simulink model "one_bot_form1"  (R2016b)
settings: Solver=ode3  StartTime=0.0  StopTime=1000  FixedStep=0.2  RelTol=1e-3  EnableMultiTasking=on
undefined symbols (not defined in the file): Angular, Linear
libraries: robotlib x7, simulink x6, realtime_pacer_lib x2
settings Model: Creator=The MathWorks Inc.  LastModifiedBy=esther
settings DataIOCC: LimitDataPoints=on  SaveFormat=Array
settings OptimizationCC: LifeSpan=Inf  MaxStackSize=64
settings DebuggingCC: SolverPrmCheckMsg=warning  SFUnexpectedBacktrackingDiag=warning  SFNoUnconditionalDefaultTransitionDiag=warning  SFExecutionAtInitializationDiag=none
settings HardwareCC: ProdBitPerPointer=32  ProdBitPerSizeT=32  ProdBitPerPtrDiffT=32  ProdLargestAtomicFloat=None  ProdIntDivRoundTo=Undefined  ProdEndianess=Unspecified  ProdWordSize=32  ProdHWDeviceType=Generic->Unspecified (assume 32-bit Generic)  TargetHWDeviceType=Generic->Unspecified (assume 32-bit Generic)
settings ModelReferenceCC: PropagateSignalLabelsOutOfModel=off
settings RTWCC: SystemTargetFile=ert.tlc  HardwareBoard=Robot Operating System (ROS)  TLCOptions=-aInlineSetEventsForThisBaseRateFcn=TLC_FALSE -aSuppressMultiTaskScheduler=TLC_FALSE -aRateBasedStepFcn=0  TemplateMakefile=ert_default_tmf  Description=Embedded Coder  Toolchain=Catkin  TargetLang=C++
settings ERTTargetCC: MultiInstanceERTCode=on  CodeInterfacePackaging=C++ class  SupportContinuousTime=on  RootIOFormat=Structure reference  ConvertIfToSwitch=off  SuppressUnreachableDefaultCases=off
settings ConfigComp: CovMetricSettings=dw  CovHtmlReporting=on  CovSaveCumulativeToWorkspaceVar=on  CovSaveSingleToWorkspaceVar=on  CovExternalEMLEnable=off  CovSFcnEnable=off

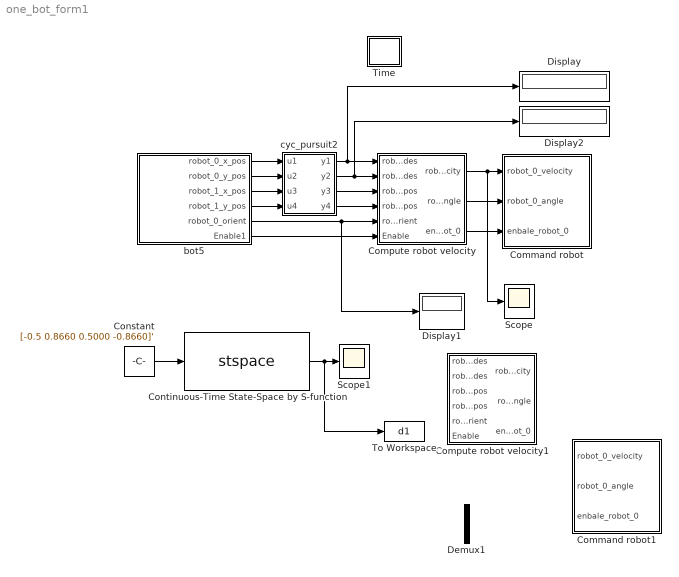
== system one_bot_form1 ==
  Command robot : Subsystem
  Command robot1 : Subsystem
  Compute robot velocity : Subsystem
  Compute robot velocity1 : Subsystem
  Constant : Constant  Value=[-0.5 0.8660 0.5000 -0.8660]'  SampleTime=-1
  Continuous-Time State-Space by S-function : S-Function  FunctionName=stspace  Parameters=a,b,c,d,x0  SFunctionDeploymentMode=off  EnableBusSupport=off  mask(S-function: stspace){a=[-1 0 1 0; 0 -1 0 1; 0 0 -1 0; 0 0 0 -1], b=eye(4), c=eye(4), d=eye(4), x0=[-0.581 -0.324 -2.225 0.735]'}
      mask prompts: x0 "Initial condition:"
      mask help: This is a S-function block which is the state-space system with dynamic inputs, outputs and states.
      mask Display: disp('dx/dt = A*X + B*U\n Y      = C*X + D*U ');
  Demux1 : Demux  Outputs=6
  Display : Display
  Display1 : Display
  Display2 : Display
  Scope : Scope
  Scope1 : Scope
  Time : Subsystem
  To Workspace : ToWorkspace  VariableName=d1  SampleTime=-1
  bot5 : Subsystem
  cyc_pursuit2 : MATLAB Function  TreatAsAtomicUnit=on
  wires:
  bot5/1(robot_0_x_pos) -> cyc_pursuit2/1(u1)
  bot5/2(robot_0_y_pos) -> cyc_pursuit2/2(u2)
  bot5/3(robot_1_x_pos) -> cyc_pursuit2/3(u3)
  bot5/4(robot_1_y_pos) -> cyc_pursuit2/4(u4)
  cyc_pursuit2/1(y1) -> Display/1, Compute robot velocity/1(robot_0_x_des)
  cyc_pursuit2/2(y2) -> Display2/1, Compute robot velocity/2(robot_0_y_des)
  cyc_pursuit2/3(y3) -> Compute robot velocity/3(robot_1_x_pos)
  cyc_pursuit2/4(y4) -> Compute robot velocity/4(robot_1_y_pos)
  Compute robot velocity/1(robot_0_velocity) -> Scope/1, Command robot/1(robot_0_velocity)
  Compute robot velocity/2(robot_0_angle) -> Command robot/2(robot_0_angle)
  Compute robot velocity/3(enable_robot_0) -> Command robot/3(enbale_robot_0)
  bot5/6(Enable1) -> Compute robot velocity/6(Enable)
  bot5/5(robot_0_orient) -> Display1/1, Compute robot velocity/5(robot_0_orient)
  Constant/1 -> Continuous-Time State-Space by S-function/1
  Continuous-Time State-Space by S-function/1 -> To Workspace/1, Scope1/1

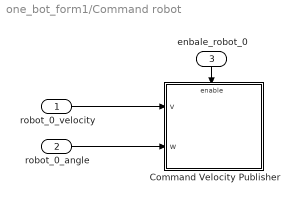
== system one_bot_form1/Command robot ==
  robot_0_velocity : Inport
  robot_0_angle : Inport  Port=2
  enbale_robot_0 : Inport  Port=3
  Command Velocity Publisher : Subsystem
  wires:
  robot_0_angle/1 -> Command Velocity Publisher/2(w)
  enbale_robot_0/1 -> Command Velocity Publisher/Enable
  robot_0_velocity/1 -> Command Velocity Publisher/1(v)

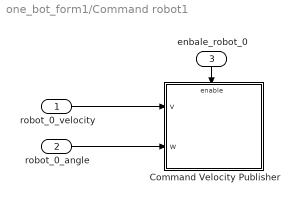
== system one_bot_form1/Command robot1 ==
  robot_0_velocity : Inport
  robot_0_angle : Inport  Port=2
  enbale_robot_0 : Inport  Port=3
  Command Velocity Publisher : Subsystem
  wires:
  robot_0_angle/1 -> Command Velocity Publisher/2(w)
  enbale_robot_0/1 -> Command Velocity Publisher/Enable
  robot_0_velocity/1 -> Command Velocity Publisher/1(v)

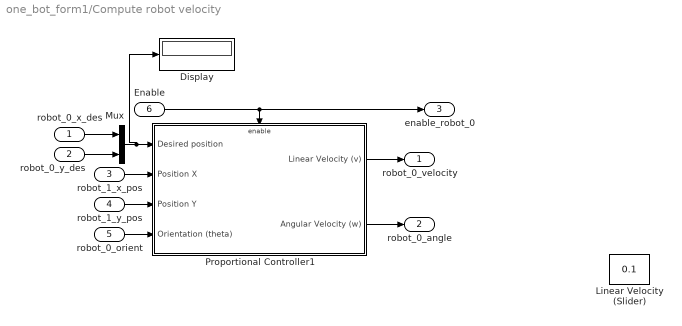
== system one_bot_form1/Compute robot velocity ==
  robot_0_x_des : Inport
  robot_0_y_des : Inport  Port=2
  robot_1_x_pos : Inport  Port=3
  robot_1_y_pos : Inport  Port=4
  robot_0_orient : Inport  Port=5
  Enable : Inport  Port=6
  Display : Display
  Linear Velocity (Slider) : simulink/Math Operations/Slider Gain  low=0  gain=0.1  high=0.2
  Mux : Mux  Inputs=2
  Proportional Controller1 : Subsystem
  robot_0_velocity : Outport
  robot_0_angle : Outport  Port=2
  enable_robot_0 : Outport  Port=3
  wires:
  Proportional Controller1/1(Linear Velocity (v)) -> robot_0_velocity/1
  Proportional Controller1/2(Angular Velocity (w)) -> robot_0_angle/1
  robot_1_x_pos/1 -> Proportional Controller1/2(Position X)
  robot_0_orient/1 -> Proportional Controller1/4(Orientation (theta))
  robot_0_x_des/1 -> Mux/1
  robot_1_y_pos/1 -> Proportional Controller1/3(Position Y)
  robot_0_y_des/1 -> Mux/2
  Enable/1 -> Proportional Controller1/Enable, enable_robot_0/1
  Mux/1 -> Display/1, Proportional Controller1/1(Desired position)

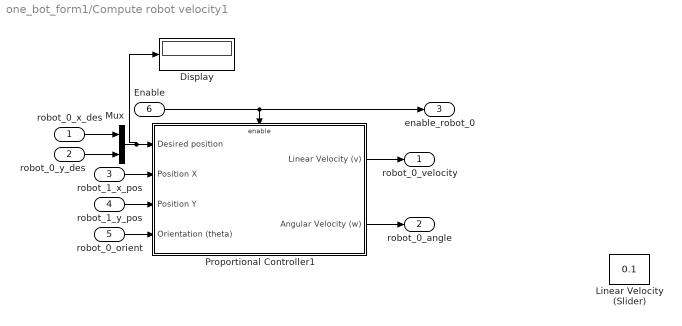
== system one_bot_form1/Compute robot velocity1 ==
  robot_0_x_des : Inport
  robot_0_y_des : Inport  Port=2
  robot_1_x_pos : Inport  Port=3
  robot_1_y_pos : Inport  Port=4
  robot_0_orient : Inport  Port=5
  Enable : Inport  Port=6
  Display : Display
  Linear Velocity (Slider) : simulink/Math Operations/Slider Gain  low=0  gain=0.1  high=0.2
  Mux : Mux  Inputs=2
  Proportional Controller1 : Subsystem
  robot_0_velocity : Outport
  robot_0_angle : Outport  Port=2
  enable_robot_0 : Outport  Port=3
  wires:
  Proportional Controller1/1(Linear Velocity (v)) -> robot_0_velocity/1
  Proportional Controller1/2(Angular Velocity (w)) -> robot_0_angle/1
  robot_1_x_pos/1 -> Proportional Controller1/2(Position X)
  robot_0_orient/1 -> Proportional Controller1/4(Orientation (theta))
  robot_0_x_des/1 -> Mux/1
  robot_1_y_pos/1 -> Proportional Controller1/3(Position Y)
  robot_0_y_des/1 -> Mux/2
  Enable/1 -> Proportional Controller1/Enable, enable_robot_0/1
  Mux/1 -> Display/1, Proportional Controller1/1(Desired position)

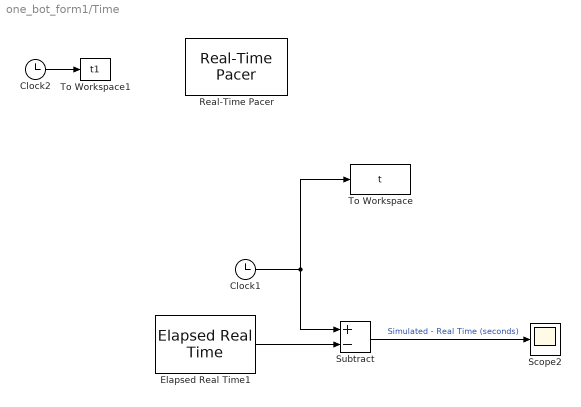
== system one_bot_form1/Time ==
  Clock1 : Clock
  Clock2 : Clock
  Elapsed Real Time1 : realtime_pacer_lib/Elapsed Real Time
  Real-Time Pacer : realtime_pacer_lib/Real-Time Pacer  simTimePerRealTime=1
  Scope2 : Scope
  Subtract : Sum  Inputs=+-
  To Workspace : ToWorkspace  VariableName=t  SaveFormat=Timeseries  SampleTime=-1
  To Workspace1 : ToWorkspace  VariableName=t1  SampleTime=-1
  wires:
  Elapsed Real Time1/1 -> Subtract/2
  Subtract/1 -> Scope2/1  "Simulated - Real Time (seconds)"
  Clock1/1 -> To Workspace/1, Subtract/1
  Clock2/1 -> To Workspace1/1

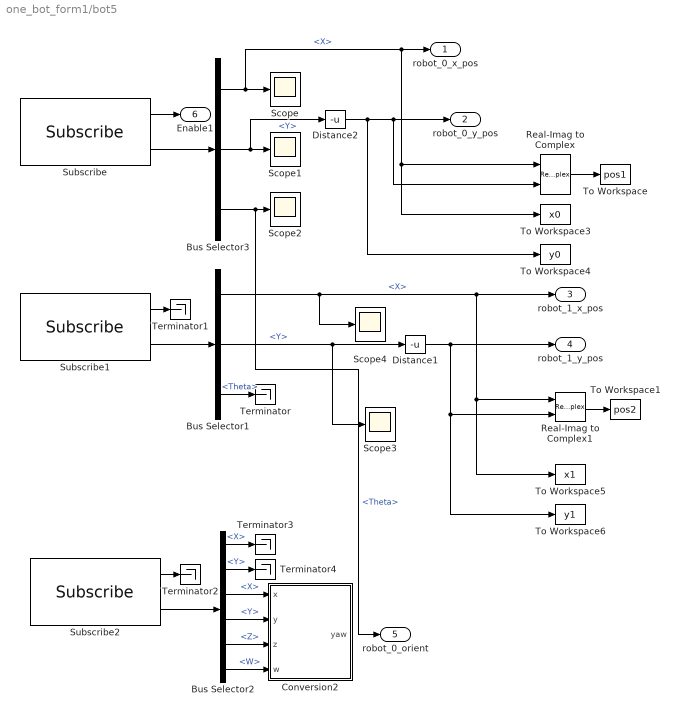
== system one_bot_form1/bot5 ==
  Bus Selector1 : BusSelector  OutputSignals=X,Y,Theta
  Bus Selector2 : BusSelector  OutputSignals=Pose.Pose.Position.X,Pose.Pose.Position.Y,Pose.Pose.Orientation.X,Pose.Pose.Orientation.Y,Pose.Pose.Orientation.Z,Pose.Pose.Orientation.W
  Bus Selector3 : BusSelector  OutputSignals=X,Y,Theta
  Conversion2 : MATLAB Function  TreatAsAtomicUnit=on
  Distance1 : Fcn  Expr=-u
  Distance2 : Fcn  Expr=-u
  Real-Imag to Complex : RealImagToComplex
  Real-Imag to Complex1 : RealImagToComplex
  Scope{,1..4} (5 alike) : Scope
  Subscribe : robotlib/Subscribe  SourceLibraryInfo=This block requires Robotics System Toolbox  topicSource=Select from ROS network  topic=/bot_0/ground_pose  messageType=geometry_msgs/Pose2D  sampleTime=-1  messageQueueLength=51
  Subscribe1 : robotlib/Subscribe  SourceLibraryInfo=This block requires Robotics System Toolbox  topicSource=Select from ROS network  topic=/bot_1/ground_pose  messageType=geometry_msgs/Pose2D  sampleTime=-1  messageQueueLength=1
  Subscribe2 : robotlib/Subscribe  SourceLibraryInfo=This block requires Robotics System Toolbox  topicSource=Select from ROS network  topic=/robot_0/pose  messageType=nav_msgs/Odometry  sampleTime=-1  messageQueueLength=1
  Terminator{,1..4} (5 alike) : Terminator
  To Workspace : ToWorkspace  VariableName=pos1  SampleTime=-1
  To Workspace1 : ToWorkspace  VariableName=pos2  SampleTime=-1
  To Workspace3 : ToWorkspace  VariableName=x0  SampleTime=-1
  To Workspace4 : ToWorkspace  VariableName=y0  SampleTime=-1
  To Workspace5 : ToWorkspace  VariableName=x1  SampleTime=-1
  To Workspace6 : ToWorkspace  VariableName=y1  SampleTime=-1
  robot_0_x_pos : Outport
  robot_0_y_pos : Outport  Port=2
  robot_1_x_pos : Outport  Port=3
  robot_1_y_pos : Outport  Port=4
  robot_0_orient : Outport  Port=5
  Enable1 : Outport  Port=6
  wires:
  Subscribe/2 -> Bus Selector3/1
  Bus Selector3/1 -> To Workspace3/1, Real-Imag to Complex/1, robot_0_x_pos/1, Scope/1  "<X>"
  Bus Selector3/2 -> Distance2/1, Scope1/1  "<Y>"
  Bus Selector3/3 -> robot_0_orient/1, Scope2/1  "<Theta>"
  Bus Selector1/1 -> Scope4/1, To Workspace5/1, Real-Imag to Complex1/1, robot_1_x_pos/1  "<X>"
  Bus Selector1/2 -> Scope3/1, Distance1/1  "<Y>"
  Subscribe1/2 -> Bus Selector1/1
  Subscribe/1 -> Enable1/1
  Subscribe1/1 -> Terminator1/1
  Real-Imag to Complex/1 -> To Workspace/1
  Real-Imag to Complex1/1 -> To Workspace1/1
  Bus Selector1/3 -> Terminator/1  "<Theta>"
  Subscribe2/2 -> Bus Selector2/1
  Bus Selector2/3 -> Conversion2/1(x)  "<X>"
  Bus Selector2/4 -> Conversion2/2(y)  "<Y>"
  Bus Selector2/5 -> Conversion2/3(z)  "<Z>"
  Subscribe2/1 -> Terminator2/1
  Bus Selector2/1 -> Terminator3/1  "<X>"
  Bus Selector2/2 -> Terminator4/1  "<Y>"
  Bus Selector2/6 -> Conversion2/4(w)  "<W>"
  Distance2/1 -> To Workspace4/1, robot_0_y_pos/1, Real-Imag to Complex/2
  Distance1/1 -> To Workspace6/1, Real-Imag to Complex1/2, robot_1_y_pos/1

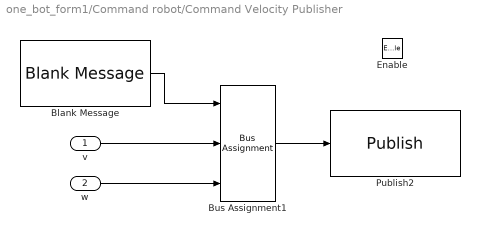
== system one_bot_form1/Command robot/Command Velocity Publisher ==
  v : Inport
  w : Inport  Port=2
  Enable : EnablePort
  Blank Message : robotlib/Blank Message  SourceLibraryInfo=This block requires Robotics System Toolbox  messageType=geometry_msgs/Twist  SampleTime=inf
  Bus Assignment1 : BusAssignment  DialogController=Simulink.DDGSource_BusAssignment  AssignedSignals=Linear.X,Angular.Z
  Publish2 : robotlib/Publish  SourceLibraryInfo=This block requires Robotics System Toolbox  topicSource=Select from ROS network  topic=/robot_0/cmd_vel  messageType=geometry_msgs/Twist  messageQueueLength=105
  wires:
  Bus Assignment1/1 -> Publish2/1
  Blank Message/1 -> Bus Assignment1/1
  v/1 -> Bus Assignment1/2
  w/1 -> Bus Assignment1/3

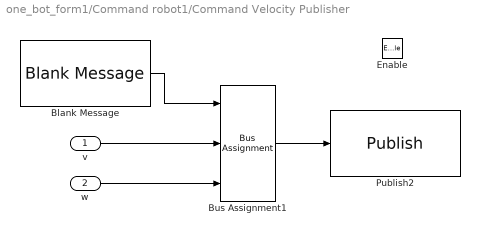
== system one_bot_form1/Command robot1/Command Velocity Publisher ==
  v : Inport
  w : Inport  Port=2
  Enable : EnablePort
  Blank Message : robotlib/Blank Message  SourceLibraryInfo=This block requires Robotics System Toolbox  messageType=geometry_msgs/Twist  SampleTime=inf
  Bus Assignment1 : BusAssignment  DialogController=Simulink.DDGSource_BusAssignment  AssignedSignals=Linear.X,Angular.Z
  Publish2 : robotlib/Publish  SourceLibraryInfo=This block requires Robotics System Toolbox  topicSource=Select from ROS network  topic=/robot_0/cmd_vel  messageType=geometry_msgs/Twist  messageQueueLength=105
  wires:
  Bus Assignment1/1 -> Publish2/1
  Blank Message/1 -> Bus Assignment1/1
  v/1 -> Bus Assignment1/2
  w/1 -> Bus Assignment1/3

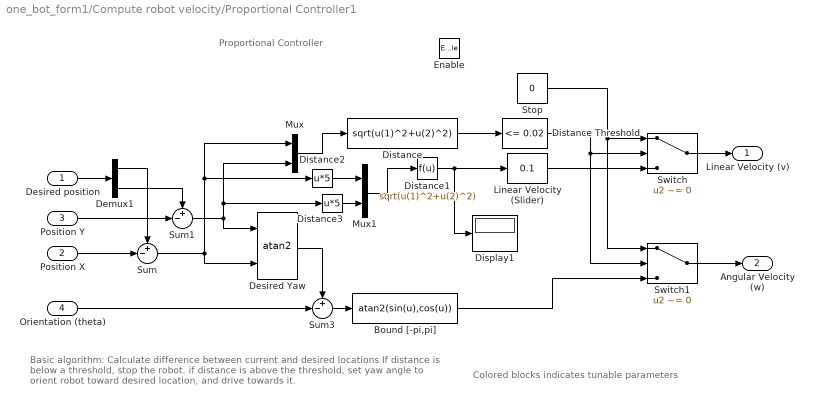
== system one_bot_form1/Compute robot velocity/Proportional Controller1 ==
  note: Proportional Controller
  note: Basic algorithm:
      | Calculate difference between current and desired locations
      | If distance is below a threshold, stop the robot.
      | if distance is above the threshold, set yaw angle to orient robot toward desired location, and drive towards it.
  note: Colored blocks indicates tunable parameters
  Desired position : Inport
  Position X : Inport  Port=2
  Position Y : Inport  Port=3
  Orientation (theta) : Inport  Port=4
  Enable : EnablePort
  Bound [-pi,pi] : Fcn  Expr=atan2(sin(u),cos(u))
  Demux1 : Demux  Outputs=2
  Desired Yaw : Trigonometry  Operator=atan2
  Display1 : Display
  Distance : Fcn  Expr=sqrt(u(1)^2+u(2)^2)
  Distance Threshold : simulink/Logic and Bit Operations/Compare To Constant  relop=<=  const=0.02  OutDataTypeStr=boolean
  Distance1 : Fcn  Expr=sqrt(u(1)^2+u(2)^2)
  Distance2 : Fcn  Expr=u*5
  Distance3 : Fcn  Expr=u*5
  Linear Velocity (Slider) : simulink/Math Operations/Slider Gain  low=0  gain=0.1  high=0.2
  Mux : Mux  Inputs=2
  Mux1 : Mux  Inputs=2
  Stop : Constant  Value=0
  Sum : Sum  Inputs=+-|
  Sum1 : Sum  Inputs=+-|
  Sum3 : Sum  Inputs=+-|
  Switch : Switch  Criteria=u2 ~= 0
  Switch1 : Switch  Criteria=u2 ~= 0
  Linear Velocity (v) : Outport
  Angular Velocity (w) : Outport  Port=2
  wires:
  Demux1/1 -> Sum/1
  Demux1/2 -> Sum1/1
  Desired position/1 -> Demux1/1
  Position Y/1 -> Sum1/2
  Position X/1 -> Sum/2
  Distance/1 -> Distance Threshold/1
  Mux/1 -> Distance/1
  Orientation (theta)/1 -> Sum3/2
  Desired Yaw/1 -> Sum3/1
  Sum/1 -> Desired Yaw/2, Distance2/1, Mux/1
  Distance Threshold/1 -> Switch/2, Switch1/2
  Bound [-pi,pi]/1 -> Switch1/3
  Stop/1 -> Switch/1, Switch1/1
  Sum3/1 -> Bound [-pi,pi]/1
  Switch/1 -> Linear Velocity (v)/1
  Linear Velocity (Slider)/1 -> Switch/3
  Switch1/1 -> Angular Velocity (w)/1
  Mux1/1 -> Distance1/1
  Distance1/1 -> Linear Velocity (Slider)/1, Display1/1
  Distance2/1 -> Mux1/1
  Distance3/1 -> Mux1/2
  Sum1/1 -> Desired Yaw/1, Mux/2, Distance3/1

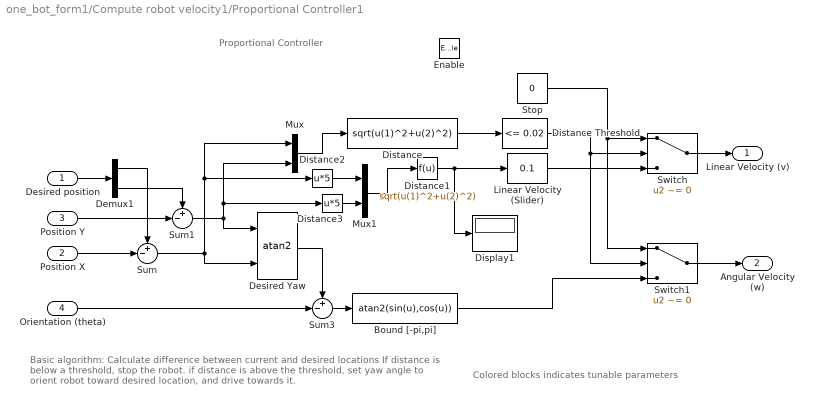
== system one_bot_form1/Compute robot velocity1/Proportional Controller1 ==
  note: Proportional Controller
  note: Basic algorithm:
      | Calculate difference between current and desired locations
      | If distance is below a threshold, stop the robot.
      | if distance is above the threshold, set yaw angle to orient robot toward desired location, and drive towards it.
  note: Colored blocks indicates tunable parameters
  Desired position : Inport
  Position X : Inport  Port=2
  Position Y : Inport  Port=3
  Orientation (theta) : Inport  Port=4
  Enable : EnablePort
  Bound [-pi,pi] : Fcn  Expr=atan2(sin(u),cos(u))
  Demux1 : Demux  Outputs=2
  Desired Yaw : Trigonometry  Operator=atan2
  Display1 : Display
  Distance : Fcn  Expr=sqrt(u(1)^2+u(2)^2)
  Distance Threshold : simulink/Logic and Bit Operations/Compare To Constant  relop=<=  const=0.02  OutDataTypeStr=boolean
  Distance1 : Fcn  Expr=sqrt(u(1)^2+u(2)^2)
  Distance2 : Fcn  Expr=u*5
  Distance3 : Fcn  Expr=u*5
  Linear Velocity (Slider) : simulink/Math Operations/Slider Gain  low=0  gain=0.1  high=0.2
  Mux : Mux  Inputs=2
  Mux1 : Mux  Inputs=2
  Stop : Constant  Value=0
  Sum : Sum  Inputs=+-|
  Sum1 : Sum  Inputs=+-|
  Sum3 : Sum  Inputs=+-|
  Switch : Switch  Criteria=u2 ~= 0
  Switch1 : Switch  Criteria=u2 ~= 0
  Linear Velocity (v) : Outport
  Angular Velocity (w) : Outport  Port=2
  wires:
  Demux1/1 -> Sum/1
  Demux1/2 -> Sum1/1
  Desired position/1 -> Demux1/1
  Position Y/1 -> Sum1/2
  Position X/1 -> Sum/2
  Distance/1 -> Distance Threshold/1
  Mux/1 -> Distance/1
  Orientation (theta)/1 -> Sum3/2
  Desired Yaw/1 -> Sum3/1
  Sum/1 -> Desired Yaw/2, Distance2/1, Mux/1
  Distance Threshold/1 -> Switch/2, Switch1/2
  Bound [-pi,pi]/1 -> Switch1/3
  Stop/1 -> Switch/1, Switch1/1
  Sum3/1 -> Bound [-pi,pi]/1
  Switch/1 -> Linear Velocity (v)/1
  Linear Velocity (Slider)/1 -> Switch/3
  Switch1/1 -> Angular Velocity (w)/1
  Mux1/1 -> Distance1/1
  Distance1/1 -> Linear Velocity (Slider)/1, Display1/1
  Distance2/1 -> Mux1/1
  Distance3/1 -> Mux1/2
  Sum1/1 -> Desired Yaw/1, Mux/2, Distance3/1

== matlab function one_bot_form1/cyc_pursuit2 ==
  data: u1 input; y1 output; u2 input; u3 input; u4 input; y2 output; y3 output; y4 output
function [y1, y2, y3, y4] = fcn(u1, u2, u3, u4)
%#codegen

y1 = ((1-0.2)*u1+(u3*0.2)-(1*0.2));
y2 = ((1-0.2)*u2+(0.2*u4)+(1.73*0.2));
y3=u1;
y4=u2;




%         y1 = ((1-0.2)*u1+(u3*0.2)+(1.5451*0.2));
%         y2 = ((1-0.2)*u2+(0.2*u4)+(4.7553*0.2));
%         y3 = ((1-0.2)*u3+(u5*0.2)-(4.0451*0.2));
%         y4 = ((1-0.2)*u4+(u6*0.2)+(2.9389*0.2));
%         y5 = ((1-0.2)*u5+(u7*0.2)-(4.0451*0.2));
%         y6 = ((1-0.2)*u6+(u8*0.2)-(2.9389*0.2));
%         y7 = ((1-0.2)*u7+(u9*0.2)+(1.5451*0.2));
%         y8 = ((1-0.2)*u8+(u10*0.2)-(4.7553*0.2));
%         y9 = ((1-0.2)*u9+(u1*0.2)+(5*0.2));
%         y10 = ((1-0.2)*u10+(u2*0.2)+(0*0.2));

== matlab function one_bot_form1/bot5/Conversion2 ==
  data: yaw output; x input; y input; z input; w input
function yaw  = quat2eul(x,y,z,w)
%#codegen

% Convert the quaternion to a yaw angle (zyx euler angle)
eul = quat2eul([w,x,y,z]);
yaw = eul(1);

end
